simulink model "FOC_PIL_Algth_top"  (R2026a)
settings: Solver=FixedStepAuto  StopTime=4  FixedStep=6.25e-5
undefined symbols (not defined in the file or in its folder): McInput_Default, McPlant_Params
settings Model: DataDictionary=McData.sldd  Creator=k  LastModifiedBy=k
settings OptimizationCC: UseDivisionForNetSlopeComputation=on  GainParamInheritBuiltInType=on  UseFloatMulNetSlope=on  InlineInvariantSignals=on  NoFixptDivByZeroProtection=on  EfficientFloat2IntCast=on  LifeSpan=1
settings RTWCC: SystemTargetFile=ert.tlc  GenerateReport=on  IncludeHyperlinkInReport=on  GenerateTraceInfo=on  GenerateTraceReport=on  GenerateTraceReportSl=on  GenerateTraceReportSf=on  GenerateTraceReportEml=on  GenerateCodeMetricsReport=on  Description=Embedded Coder
settings ERTTargetCC: GenerateSampleERTMain=on  IncludeMdlTerminateFcn=off  CombineSignalStateStructs=on  SupportComplex=off  SupportNonInlinedSFcns=on

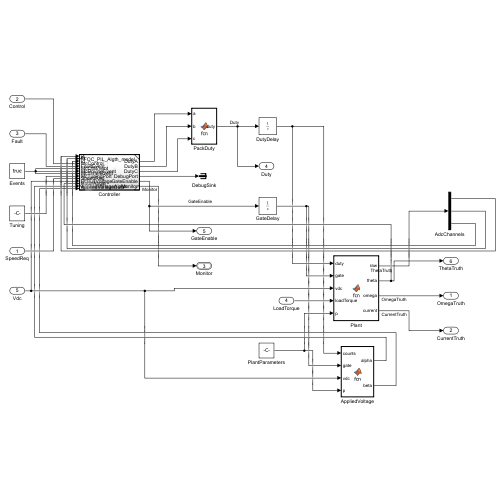
[thumbnail: Simulink's stored preview of the top-level diagram]
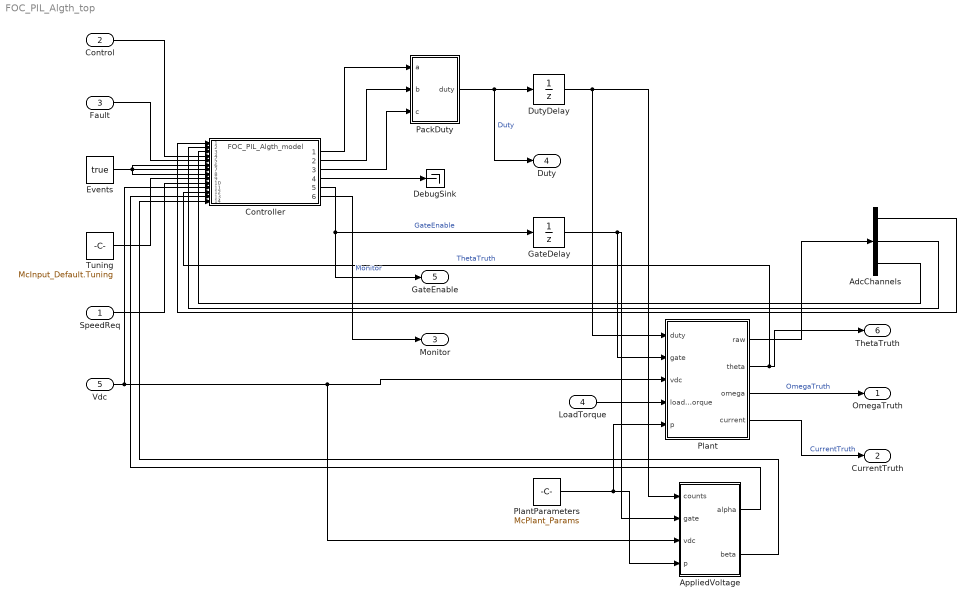
== system FOC_PIL_Algth_top ==
  SpeedReq : Inport  OutDataTypeStr=single  SampleTime=6.25e-5
  Control : Inport  Port=2  OutDataTypeStr=uint8  SampleTime=6.25e-5
  Fault : Inport  Port=3  OutDataTypeStr=boolean  SampleTime=6.25e-5
  LoadTorque : Inport  Port=4  OutDataTypeStr=double  SampleTime=6.25e-5
  Vdc : Inport  Port=5  OutDataTypeStr=single  SampleTime=6.25e-5
  AdcChannels : Demux  Outputs=3
  AppliedVoltage : MATLAB Function  TreatAsAtomicUnit=on
  Controller : ModelReference  ModelNameDialog=FOC_PIL_Algth_model  SimulationMode=Normal  ModelReferenceVersion=1.3
  DebugSink : Terminator
  DutyDelay : UnitDelay  InitialCondition=uint16([32768;32768;32768])  SampleTime=6.25e-5
  Events : Constant  Value=true  OutDataTypeStr=boolean
  GateDelay : UnitDelay  InitialCondition=false  SampleTime=6.25e-5
  PackDuty : MATLAB Function  TreatAsAtomicUnit=on
  Plant : MATLAB Function  TreatAsAtomicUnit=on
  PlantParameters : Constant  Value=McPlant_Params  OutDataTypeStr=Bus: tMcControlParams
  Tuning : Constant  Value=McInput_Default.Tuning  OutDataTypeStr=Bus: tMcTuning
  OmegaTruth : Outport  OutDataTypeStr=single
  CurrentTruth : Outport  Port=2  OutDataTypeStr=single
  Monitor : Outport  Port=3  OutDataTypeStr=Bus: tMcMonitor
  Duty : Outport  Port=4  OutDataTypeStr=uint16
  GateEnable : Outport  Port=5  OutDataTypeStr=boolean
  ThetaTruth : Outport  Port=6  OutDataTypeStr=single
  wires:
  AppliedVoltage/2(beta) -> Controller/14
  AppliedVoltage/1(alpha) -> Controller/13
  Events/1 -> Controller/8, Controller/6, Controller/7
  Controller/4 -> DebugSink/1
  Controller/6 -> Monitor/1  "Monitor"
  Controller/5 -> GateDelay/1, GateEnable/1  "GateEnable"
  PackDuty/1(duty) -> DutyDelay/1, Duty/1  "Duty"
  Plant/4(current) -> CurrentTruth/1  "CurrentTruth"
  Plant/3(omega) -> OmegaTruth/1  "OmegaTruth"
  Plant/2(theta) -> ThetaTruth/1, Controller/12  "ThetaTruth"
  SpeedReq/1 -> Controller/10
  Tuning/1 -> Controller/9
  Fault/1 -> Controller/5
  Control/1 -> Controller/4
  Controller/3 -> PackDuty/3(c)
  AdcChannels/3 -> Controller/3
  Controller/2 -> PackDuty/2(b)
  AdcChannels/2 -> Controller/2
  Controller/1 -> PackDuty/1(a)
  AdcChannels/1 -> Controller/1
  Plant/1(raw) -> AdcChannels/1
  PlantParameters/1 -> Plant/5(p), AppliedVoltage/4(p)
  LoadTorque/1 -> Plant/4(loadTorque)
  Vdc/1 -> AppliedVoltage/3(vdc), Plant/3(vdc), Controller/11
  GateDelay/1 -> AppliedVoltage/2(gate), Plant/2(gate)
  DutyDelay/1 -> Plant/1(duty), AppliedVoltage/1(counts)

== matlab function FOC_PIL_Algth_top/PackDuty ==
  data: a input; duty output; b input; c input
function duty=fcn(a,b,c)
%#codegen
duty=[a;b;c];
end

== matlab function FOC_PIL_Algth_top/Plant ==
  data: duty input; raw output; gate input; vdc input; loadTorque input; p input; theta output; omega output; current output
function [raw,theta,omega,current]=fcn(duty,gate,vdc,loadTorque,p)
%#codegen
persistent x
if isempty(x),x=zeros(4,1);end
x=mc.plant_step(x,double(duty)/double(p.PwmPeriod),vdc,loadTorque,gate,p,6.25e-5);
[raw,current,theta,omega]=mc.plant_measure(x,p);
end

== matlab function FOC_PIL_Algth_top/AppliedVoltage ==
  data: counts input; alpha output; gate input; vdc input; p input; beta output
function [alpha,beta]=fcn(counts,gate,vdc,p)
%#codegen
voltage=mc.applied_voltage(counts,vdc,gate,p.PwmPeriod);
alpha=voltage(1);beta=voltage(2);
end
